simulink model "DCMG_BDCSUIO_jan2025_scenario_1"  (R2018b)
settings: Solver=ode1  StartTime=0.0  StopTime=2  FixedStep=1e-6  RelTol=1e-3
undefined symbols (not defined in the file): Cdc, dEgdT, EgRef, gcbh, k1, Rsh_array5pc, sigbuilder_block, sps_rtmsupport, Tref_K, VT_ref
libraries: powerlib x41, spsPVarrayModel x3
(part 2 of 6)

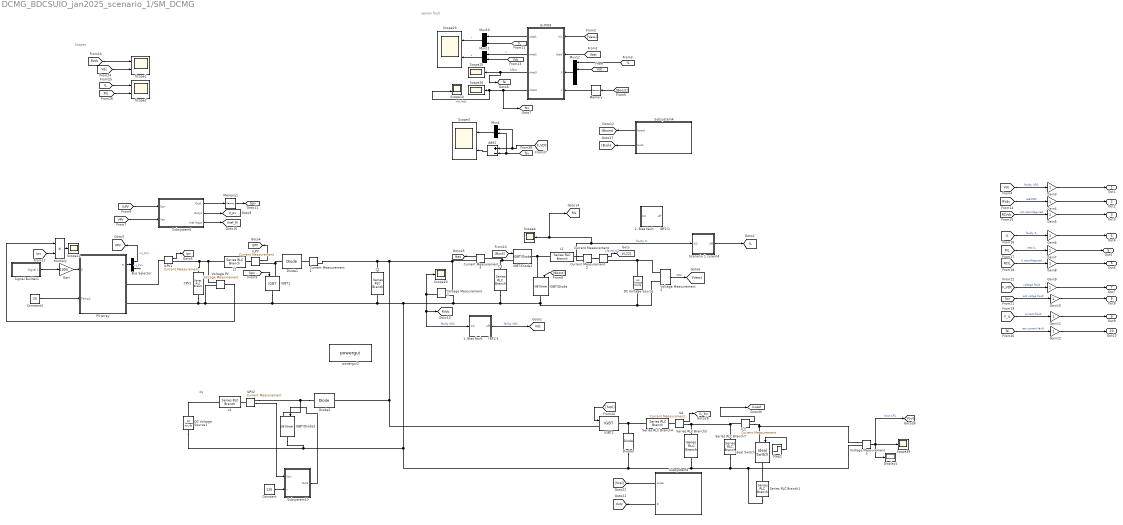
== system DCMG_BDCSUIO_jan2025_scenario_1/SM_DCMG ==
  note: Scopes
  note: dg
  note: sensor fault
  " Ui-PIO3" : MATLAB Function  TreatAsAtomicUnit=on
  1.	Bias fault      (BF1)1 : Subsystem
  2.	Bias fault      (BF2)1 : Subsystem
  Add1 : Sum  Inputs=+-
  Bus Selector : BusSelector  OutputSignals=V_PV,I_PV
  C1 : powerlib/Elements/Series RLC Branch  LConnTagsString=__new0  RConnTagsString=__new0  BranchType=R  Resistance=120  Inductance=1e-3  SetiL0=off  InitialCurrent=0  Capacitance=Cdc  Setx0=on  InitialVoltage=Vdcref  Measurements=None
      settings: SourceProductName=Simscape Electrical
  C3 : powerlib/Elements/Series RLC Branch  LConnTagsString=__new0  RConnTagsString=__new0  BranchType=C  Resistance=1e-3  Inductance=1e-3  SetiL0=off  InitialCurrent=0  Capacitance=900e-06  Setx0=on  InitialVoltage=380  Measurements=None
      settings: SourceProductName=Simscape Electrical
  CPV1 : powerlib/Elements/Series RLC Branch  LConnTagsString=__new0  RConnTagsString=__new0  BranchType=C  Resistance=1  Inductance=1e-3  SetiL0=off  InitialCurrent=0  Capacitance=35e-6  Setx0=off  InitialVoltage=120  Measurements=None
  Constant : Constant  Value=120
  Constant2 : Constant  Value=25
  Current Measurement{1..3,5} (4 alike) : powerlib/Measurements/Current Measurement  PhasorSimulation=off  OutputType=Complex  PSBequivalent=0
  DC Voltage Source : powerlib/Electrical Sources/DC Voltage Source  Amplitude=160  Measurements=None
  DC Voltage Source1 : powerlib/Electrical Sources/DC Voltage Source  Amplitude=120  Measurements=None
  Diode1 : powerlib/Power Electronics/Diode  Ron=0.001  Lon=0  Vf=0.8  IC=0  UseSnubber=0  Rs=500  Cs=250e-9  Measurements=off
  Diode2 : powerlib/Power Electronics/Diode  Ron=0.001  Lon=0  Vf=0.8  IC=0  UseSnubber=0  Rs=500  Cs=250e-9  Measurements=off
  Diode3 : powerlib/Power Electronics/Diode  Ron=0.001  Lon=0  Vf=0.8  IC=0  UseSnubber=0  Rs=500  Cs=250e-9  Measurements=off
      settings: SourceProductName=Simscape Electrical
  Display1 : Display
  Gain : Gain  Gain=1000
  Gain{3..12} (10 alike) : Gain
  IGBT/Diode : powerlib/Power Electronics/IGBT//Diode  Ron=1e-3  Rs=1e5  Cs=inf  Measurements=off
  IGBT/Diode1 : powerlib/Power Electronics/IGBT//Diode  Ron=1e-3  Rs=1e5  Cs=inf  Measurements=off
  IGBT/Diode2 : powerlib/Power Electronics/IGBT//Diode  Ron=1e-3  Rs=1e5  Cs=inf  Measurements=off
  IGBT1 : powerlib/Power Electronics/IGBT  Ron=0.001  Lon=0  Vf=1  Tf=1e-6  Tt=2e-6  IC=0  Rs=1e5  Cs=inf  Measurements=off
  IGBT2 : powerlib/Power Electronics/IGBT  Ron=0.001  Lon=0  Vf=1  Tf=1e-6  Tt=2e-6  IC=0  Rs=1e5  Cs=inf  Measurements=off
      settings: SourceProductName=Simscape Electrical
  IL2 : powerlib/Measurements/Current Measurement  PhasorSimulation=off  OutputType=Complex  PSBequivalent=0
      settings: SourceProductName=Simscape Electrical
  IL4 : powerlib/Measurements/Current Measurement  PhasorSimulation=off  OutputType=Complex  PSBequivalent=0
      settings: SourceProductName=Simscape Electrical
  ILPV : powerlib/Measurements/Current Measurement  PhasorSimulation=off  OutputType=Complex  PSBequivalent=0
  ILPV1 : powerlib/Measurements/Current Measurement  PhasorSimulation=off  OutputType=Complex  PSBequivalent=0
  ILPV2 : powerlib/Measurements/Current Measurement  PhasorSimulation=off  OutputType=Complex  PSBequivalent=0
  Ideal Switch : powerlib/Power Electronics/Ideal Switch  Ron=0.001  Lon=0  IC=0  Rs=1e5  Cs=inf  Measurements=off
  L1 : powerlib/Elements/Series RLC Branch  LConnTagsString=__new0  RConnTagsString=__new0  BranchType=RL  Resistance=0.016  Inductance=0.012  SetiL0=off  InitialCurrent=0  Capacitance=1e-6  Setx0=off  InitialVoltage=0  Measurements=None
      settings: SourceProductName=Simscape Electrical
  L2 : powerlib/Elements/Series RLC Branch  LConnTagsString=__new0  RConnTagsString=__new0  BranchType=RL  Resistance=0.09  Inductance=0.019  SetiL0=off  InitialCurrent=0  Capacitance=1e-6  Setx0=off  InitialVoltage=0  Measurements=None
  L3 : powerlib/Elements/Series RLC Branch  LConnTagsString=__new0  RConnTagsString=__new0  BranchType=RL  Resistance=0.016  Inductance=0.012  SetiL0=off  InitialCurrent=0  Capacitance=1e-6  Setx0=off  InitialVoltage=0  Measurements=None
  Memory : Memory
  Memory1 : Memory
  Multiply : Product
  Mux1 : Mux  Inputs=2
  Mux10 : Mux  Inputs=2
  Mux11 : Mux  Inputs=2
  Mux12 : Mux
  PV Array : Subsystem  AncestorBlock=re_lib/Solar/PV Array  DialogController=POWERSYS.PowerSysDialog  LoadFcn=sps_rtmsupport('LoadFcn',gcbh);  StartFcn=sps_rtmsupport('StartFcn',gcbh);  StopFcn=sps_rtmsupport('StopFcn',gcbh);  mask(PV array){Npar=5, Nser=4, PlotType=array @ 25 deg.C & specified irradiances, S_vec=[ 1000  500  100 ], Temp_C_vec=[ 45 25  ], ModuleName=BP Solar BP3175N, PlotWhenSelected=off, Pm=174.44, Ncell=72, Voc=43.6, Isc=5.3, Vm=35.6, Im=4.9, beta_Voc_pc=-0.39851, alpha_Isc_pc=0.1136, beta_Voc=-0.17375, alpha_Isc=0.006021, IL=5.317, I0=6.8296e-10, nI=1.0363, Rsh=263.997, Rs=0.48703, BAL=off, Tc=1e-6, Tfilter=5e-5}
      mask prompts: Npar "Parallel strings"; Nser "Series-connected modules per string"; S_vec "Irradiances (W/m2)"; Temp_C_vec "T_cell (deg. C)"; ModuleName "Module:"; PlotWhenSelected "Plot I-V and P-V characteristics when a module is selected"; Pm "Maximum Power (W)"; Ncell "Cells per module (Ncell)"; Voc "Open circuit voltage  Voc (V)"; Isc "Short-circuit current Isc (A)"; Vm "Voltage at maximum power point Vmp (V)"; Im "Current at maximum power point Imp (A)"; beta_Voc_pc "Temperature coefficient of Voc (%/deg.C)"; alpha_Isc_pc "Temperature coefficient of Isc (%/deg.C)"; beta_Voc "Temperature coefficient of Voc (V/deg.C)"; alpha_Isc "Temperature coefficient of Isc (A/deg.C)"; IL "Light-generated current IL (A)"; I0 "Diode saturation current I0 (A)"; nI "Diode ideality factor"; Rsh "Shunt resistance Rsh (ohms)"; Rs "Series resistance Rs (ohms)"; BAL "Break algebaic loop in internal model"; Tc "Time constant (s)"; Tfilter "Time constant (s)"
      mask help:
      | Implements a PV array built of strings of PV modules connected in parallel. Each string consists of modules connected in series.
      | Allows modeling of a variety of preset PV modules available from NREL System Advisor Model (Jan. 2014) as well as user-defined PV module.
      |
      | Input 1 = Sun irradiance, in W/m2, and input 2 = Cell temperature, in deg.C.
      mask init:
      | Block = gcb;
      | [k,k1,q,Tref_C,Tref_K,EgRef,dEgdT,Rsh_array5pc,VT_ref,Tsf,Tf,WantBlockChoice] = PVArrayInit(Block, ModuleName, Nser, Npar, Ncell, Rsh, nI, Tfilter);
      | powericon('SetInternalModels','set',Block,WantBlockChoice);
      | sps_rtmsupport('parametereditingmodes',Block, [3 6 7 23]);
      settings: CopyFcn=sps_rtmsupport('CopyFcn',gcbh);  DeleteFcn=sps_rtmsupport('DeleteFcn',gcbh);  UndoDeleteFcn=sps_rtmsupport('UndoDeleteFcn',gcbh);  ModelCloseFcn=sps_rtmsupport('ModelCloseFcn',gcbh);  PreSaveFcn=sps_rtmsupport('PreSaveFcn',gcbh);  PostSaveFcn=sps_rtmsupport('PostSaveFcn',gcbh);  NameChangeFcn=sps_rtmsupport('NameChangeFcn',gcbh);  PreCopyFcn=sps_rtmsupport('PreCopyFcn',gcbh);  CloseFcn=sps_rtmsupport('CloseFcn',gcbh);  PreDeleteFcn=sps_rtmsupport('PreDeleteFcn',gcbh);
      settings: OpenFcn=|
      | %assignin('base','PVMaskOpening',1);
      | %open_system(gcb,'mask')
      | %assignin('base','PVMaskOpening',0);
      | sps_rtmsupport('OpenFcn',gcbh, [3 6 7 23]);
      mask Help: helpview(psbhelp);
      mask TypeOptions PlotType: one module @ 25 deg.C & specified irradiances | array @ 25 deg.C & specified irradiances | array @ 1000 W/m2 & specified temperatures
      mask Callback PlotType: PVArrayCback(gcb)
